simulink model "ekffede"  (Simulink 7.7)
settings: Solver=ode3  StartTime=0.0  StopTime=200  FixedStep=0.01  RelTol=1e-3
undefined symbols (not defined in the file): aerosimlib, Earth, WGS, WMM
libraries: simulink x15, aerolibconvert2 x4, aerolibtransform2 x2, aerolibgravity2 x2, aerolib6dof2 x1
settings Model: Creator="Fabrizio  Giulietti"  LastModifiedBy=Fede
settings OptimizationCC: InitFltsAndDblsToZero=on  OptimizeModelRefInitCode=on  LifeSpan=1
settings DebuggingCC: StrictBusMsg=Warning
settings HardwareCC: ProdLargestAtomicInteger=Long  ProdLargestAtomicFloat=Float  ProdEndianess=LittleEndian  ProdHWDeviceType=ARM Compatible->ARM 9
settings SFSimCC: SimParseCustomCode=off
settings RTWCC: SystemTargetFile=ert.tlc  TemplateMakefile=ert_default_tmf  Description=Embedded Coder  ProcessScript=ert_make_rtw_hook  RTWCompilerOptimization=On
settings CodeAppCC: IgnoreCustomStorageClasses=off
settings ERTTargetCC: FunctionExecutionProfile=off  MultiwordLength=2048  GenerateSampleERTMain=on  ERTCustomFileTemplate=example_file_process.tlc  ConvertIfToSwitch=off

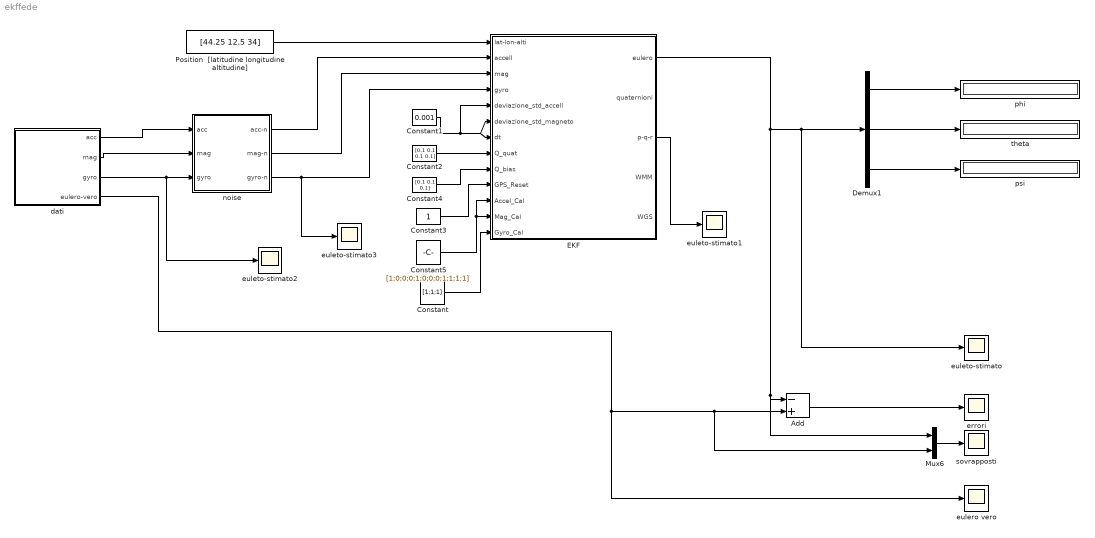
== system ekffede ==
  Add : Sum  Inputs=-+
  Constant : Constant  Value=[1;1;1]
  Constant1 : Constant  Value=0.001
  Constant2 : Constant  Value=[0.1 0.1 0.1 0.1]
  Constant3 : Constant
  Constant4 : Constant  Value=[0.1 0.1 0.1]
  Constant5 : Constant  Value=[1;0;0;0;1;0;0;0;1;1;1;1]
  Demux1 : Demux  Outputs=3
  EKF : Subsystem
  Mux6 : Mux  Inputs=2
  Position  [latitudine longitudine altitudine] : Constant  Value=[44.25 12.5 34]
  dati : Subsystem
  errori : Scope
      settings: YMin=-1.25  YMax=1.25
  eulero vero : Scope
      settings: SaveName=ScopeData15
  euleto-stimato{,1..3} (4 alike) : Scope
      euleto-stimato settings: YMin=-200  YMax=200  SaveName=ScopeData7
      euleto-stimato1 settings: YMin=-0.65  YMax=0.05  SaveName=ScopeData19
      euleto-stimato2 settings: SaveName=ScopeData20
      euleto-stimato3 settings: SaveName=ScopeData21
  noise : Subsystem  mask{bias_acc=|, bias_gyro=|, bias_mag=|, accel_noise_power=[0.0000, 0.0000, 0.0000], gyro_noise_power=[0.0000, 0.0000, 0.0000], mag_noise_power=[0.00000, 0.00000, 0.00000], acc_noise_freq=0.01, gyro_noise_freq=0.01, mag_noise_freq=0.01}
      mask bias_acc=|
      | [0  ;   0
      |  ;    0]
      mask bias_gyro=|
      | [0 ;   0
      |  ;    0]
      mask bias_mag=|
      | [0  ;   0
      |  ;    0]
      mask prompts: bias_acc "bias-acc"; bias_gyro "bias-gyro"; bias_mag "bias-mag"; accel_noise_power "accel-noise-power"; gyro_noise_power "gyro-noise-power"; mag_noise_power "mag-noise-power"; acc_noise_freq "acc-noise-freq"; gyro_noise_freq "gyro-noise-freq"; mag_noise_freq "mag-noise-freq"
  phi : Display
  psi : Display
  sovrapposti : Scope
      settings: TimeRange=200  YMin=-85  SaveName=ScopeData9
  theta : Display
  wires:
  Demux1/1 -> phi/1
  Demux1/2 -> theta/1
  Demux1/3 -> psi/1
  EKF/1(eulero) -> Demux1/1, euleto-stimato/1, Add/1, Mux6/1
  dati/4(eulero-vero) -> Add/2, Mux6/2, eulero vero/1
  Add/1 -> errori/1
  dati/2(mag) -> noise/2(mag)
  dati/3(gyro) -> noise/3(gyro), euleto-stimato2/1
  noise/2(mag-n) -> EKF/3(mag)
  Position  [latitudine longitudine altitudine]/1 -> EKF/1(lat-lon-alti)
  noise/3(gyro-n) -> EKF/4(gyro), euleto-stimato3/1
  noise/1(acc-n) -> EKF/2(accell)
  dati/1(acc) -> noise/1(acc)
  EKF/3(p-q-r) -> euleto-stimato1/1
  Constant1/1 -> EKF/5(deviazione_std_accell), EKF/6(deviazione_std_magneto), EKF/7(dt)
  Constant2/1 -> EKF/8(Q_quat)
  Constant4/1 -> EKF/9(Q_bias)
  Constant3/1 -> EKF/10(GPS_Reset)
  Mux6/1 -> sovrapposti/1
  Constant/1 -> EKF/13(Gyro_Cal)
  Constant5/1 -> EKF/11(Accel_Cal), EKF/12(Mag_Cal)

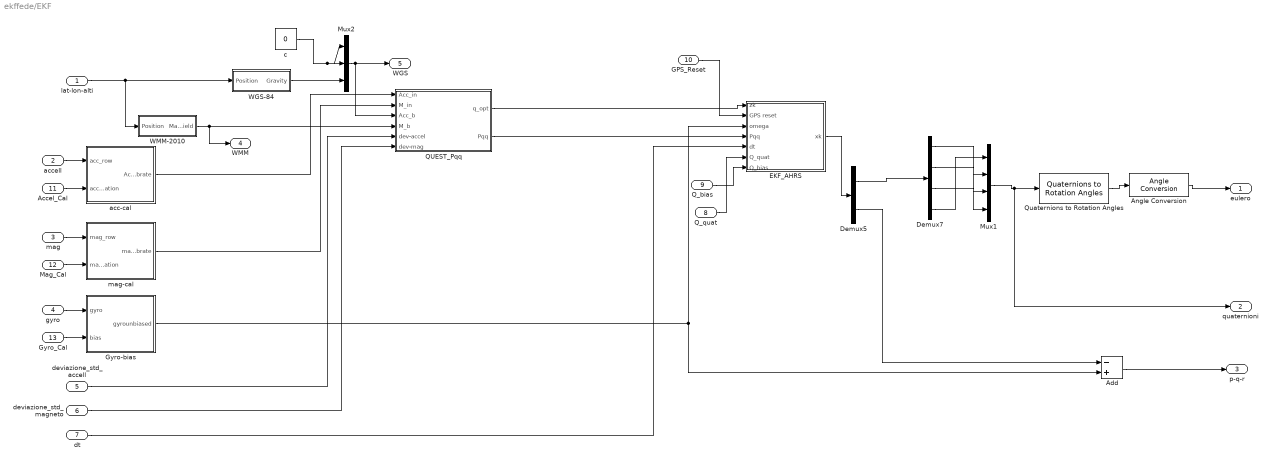
== system ekffede/EKF ==
  lat-lon-alti : Inport
  accell : Inport  Port=2  OutDataTypeStr=double
  mag : Inport  Port=3  OutDataTypeStr=double
  gyro : Inport  Port=4  OutDataTypeStr=double
  deviazione_std_accell : Inport  Port=5
  deviazione_std_magneto : Inport  Port=6
  dt : Inport  Port=7
  Q_quat : Inport  Port=8
  Q_bias : Inport  Port=9
  GPS_Reset : Inport  Port=10
  Accel_Cal : Inport  Port=11  OutDataTypeStr=double
  Mag_Cal : Inport  Port=12  OutDataTypeStr=double
  Gyro_Cal : Inport  Port=13  OutDataTypeStr=double
  Add : Sum  Inputs=-+
  Angle Conversion : aerolibconvert2/Angle Conversion  SystemSampleTime=-1  IU=rad  OU=deg
  Demux5 : Demux  Outputs=[4 3]
  Demux7 : Demux
  EKF_AHRS : Subsystem  mask{x0=[0 0 0 0 0 0 0]'}
      mask prompts: x0 "Initial condition vector"
  Gyro-bias : Stateflow chart  TreatAsAtomicUnit=on
  Mux1 : Mux
  Mux2 : Mux  Inputs=3
  QUEST_Pqq : Subsystem
  Quaternions to Rotation Angles : aerolibtransform2/Quaternions to Rotation Angles  SystemSampleTime=-1  rotationOrder=XYZ
  WGS-84 : Subsystem  AncestorBlock=aerosimlib/Earth/WGS-84
      mask Type: WGS-84 Earth model
      mask Description: The WGS-84 Earth model provides local Earth radii and gravity as a function of position.
      mask Help:
      | The block provides a WGS-84 geoid model of the Earth.
      | <P><B>Inputs:</B>
      | <LI>Position = current aircraft location [Latitude Longitude Altitude], in [rad rad m]</LI>
      | </P>
      | <P><B>Output:</B>
      | <LI>Rmeridian = the Earth meridian radius, in m</LI>
      | <LI>Rnormal = the Earth normal radius, in m</LI>
      | <LI>Re = the Earth equivalent radius, in m</LI>
      | <LI>Gravity = the normal gravity, in m/s^2</LI>
      | </P>
  WMM-2010 : Subsystem  AncestorBlock=aerosimlib/Earth/WMM-2000  mask(WMM-2000){wmmfile='C:\\Programmmi\\AeroSim\\wmm.cof', simdate=[26 05 2011]}
      mask prompts: wmmfile "WMM coefficient file:"; simdate "Simulation date [Day Month Year]:"
      mask help: The World Magnetic Model returns the Earth magnetic field components in body axes at current aircraft location.
      mask Help:
      | The block provides the magnetic field components at current aircraft location.
      | <P><B>Inputs:</B>
      | <LI>Position = the 3x1 vector of aircraft location [Latitude Longitude Altitude] in [rad rad m]</LI>
      | <LI>DCM = the frame transformation matrix from navigation to body frame</LI>
      | </P>
      | <P><B>Output:</B>
      | <LI>MagField = the 3x1 vector of magnetic field components in body axes</LI>
      | </P>
      | <P><B>Parameters:</B>
      | <LI>WMM coefficient file = the path to the WMM coefficient file, as a 'string'</LI>
      | <LI>Simulation date = the 1x3 vector of current date [Day Month Year]</LI>
      | </P>
  acc-cal : Stateflow chart  TreatAsAtomicUnit=on
  c : Constant  Value=0
  mag-cal : Stateflow chart  TreatAsAtomicUnit=on
  eulero : Outport
  quaternioni : Outport  Port=2
  p-q-r : Outport  Port=3
  WMM : Outport  Port=4
  WGS : Outport  Port=5
  wires:
  c/1 -> Mux2/1, Mux2/2
  Mux2/1 -> QUEST_Pqq/3(Acc_b), WGS/1
  lat-lon-alti/1 -> WMM-2010/1(Position), WGS-84/1(Position)
  GPS_Reset/1 -> EKF_AHRS/2(GPS reset)
  QUEST_Pqq/2(Pqq) -> EKF_AHRS/4(Pqq)
  Demux5/2 -> Add/1
  Quaternions to Rotation Angles/1 -> Angle Conversion/1
  WMM-2010/1(MagField) -> QUEST_Pqq/4(M_b), WMM/1
  WGS-84/1(Gravity) -> Mux2/3
  Angle Conversion/1 -> eulero/1
  Add/1 -> p-q-r/1
  deviazione_std_accell/1 -> QUEST_Pqq/5(dev-accel)
  deviazione_std_magneto/1 -> QUEST_Pqq/6(dev-mag)
  dt/1 -> EKF_AHRS/5(dt)
  EKF_AHRS/1(xk) -> Demux5/1
  Q_quat/1 -> EKF_AHRS/6(Q_quat)
  Q_bias/1 -> EKF_AHRS/7(Q_bias)
  Demux5/1 -> Demux7/1
  Mux1/1 -> Quaternions to Rotation Angles/1, quaternioni/1
  Demux7/4 -> Mux1/1
  Demux7/1 -> Mux1/2
  Demux7/2 -> Mux1/3
  Demux7/3 -> Mux1/4
  QUEST_Pqq/1(q_opt) -> EKF_AHRS/1(zk)
  Gyro-bias/1(gyrounbiased) -> EKF_AHRS/3(omega), Add/2
  Gyro_Cal/1 -> Gyro-bias/2(bias)
  gyro/1 -> Gyro-bias/1(gyro)
  accell/1 -> acc-cal/1(acc_row)
  acc-cal/1(Acc_calibrate) -> QUEST_Pqq/1(Acc_in)
  Accel_Cal/1 -> acc-cal/2(acc_calibration)
  Mag_Cal/1 -> mag-cal/2(mag_calibration)
  mag/1 -> mag-cal/1(mag_row)
  mag-cal/1(mag_calibrate) -> QUEST_Pqq/2(M_in)

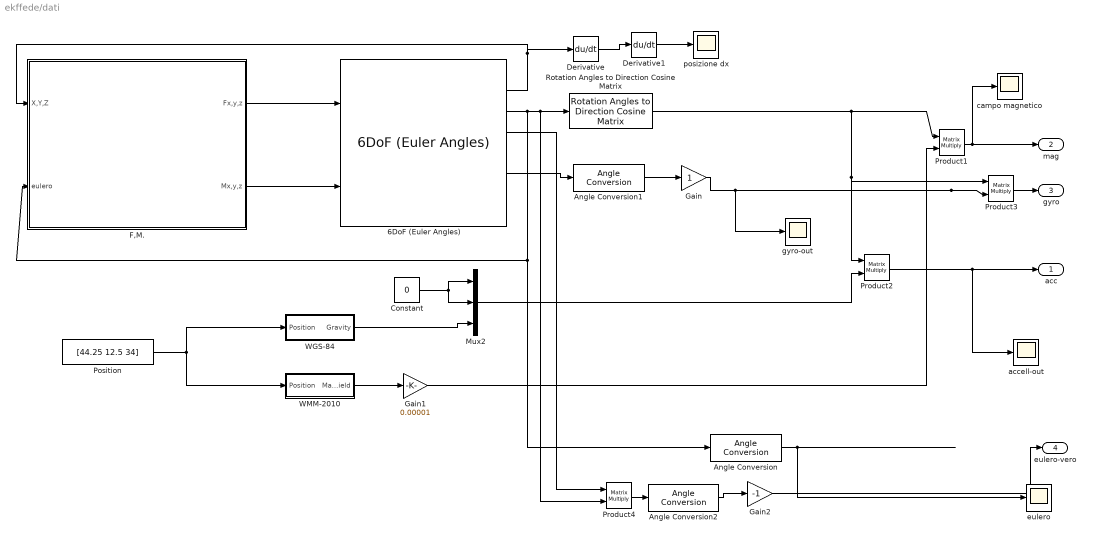
== system ekffede/dati ==
  6DoF (Euler Angles) : aerolib6dof2/6DoF (Euler Angles)  SystemSampleTime=-1  units=Metric (MKS)  mtype=Fixed  rep=Euler Angles  xme_0=[0 0 0]  Vm_0=[0 0 0]  eul_0=[0 0 0]  pm_0=[0 0 0]  mass_0=1000  mass_e=0.5  mass_f=2.0  inertia=eye(3)  inertia_e=eye(3)  inertia_f=2*eye(3)  k_quat=1.0
  Angle Conversion : aerolibconvert2/Angle Conversion  SystemSampleTime=-1  IU=rad  OU=deg
  Angle Conversion1 : aerolibconvert2/Angle Conversion  SystemSampleTime=-1  IU=rad  OU=rad
  Angle Conversion2 : aerolibconvert2/Angle Conversion  SystemSampleTime=-1  IU=rad  OU=deg
  Constant : Constant  Value=0
  Derivative : Derivative
  Derivative1 : Derivative
  F,M. : Subsystem  mask{rate_limiter_sfasamento=0.2, Fx=0, Fy=0, ampiezza_Fz=0.01, ampiezza_Fy=0, ampiezza_Fx=0, ampiezza_Mx=0.05, ampiezza_My=0.09, ampiezza_Mz=3.5, frequenza_Fz=0.01, frequenza_Fy=0.01, frequenza_Fx=0.01, frequenza_Mx=0.01, frequenza_My=0.01, frequenza_Mz=0.01, noise_power_sfasamento_m=0, sample_time_sfasamento_m=20, noise_power_m=0, noise_time_m=100, noise_power_F=0, noise_time_F=200, noise_power_sfasamento_F=0, sample_time_sfasamento_F=200}
      mask prompts: noise_power_sfasamento_F "sample_power_sfasamento_F"
  Gain : Gain
  Gain1 : Gain  Gain=0.00001
  Gain2 : Gain  Gain=-1
  Mux2 : Mux  Inputs=3
  Position : Constant  Value=[44.25 12.5 34]
  Product{1..4} (4 alike) : Product  Multiplication=Matrix(*)  RndMeth=Zero
  Rotation Angles to Direction Cosine Matrix : aerolibtransform2/Rotation Angles to Direction Cosine Matrix  SystemSampleTime=-1  rotationOrder=XYZ
  WGS-84 : Subsystem  AncestorBlock=aerosimlib/Earth/WGS-84
      mask Type: WGS-84 Earth model
      mask Description: The WGS-84 Earth model provides local Earth radii and gravity as a function of position.
      mask Help:
      | The block provides a WGS-84 geoid model of the Earth.
      | <P><B>Inputs:</B>
      | <LI>Position = current aircraft location [Latitude Longitude Altitude], in [rad rad m]</LI>
      | </P>
      | <P><B>Output:</B>
      | <LI>Rmeridian = the Earth meridian radius, in m</LI>
      | <LI>Rnormal = the Earth normal radius, in m</LI>
      | <LI>Re = the Earth equivalent radius, in m</LI>
      | <LI>Gravity = the normal gravity, in m/s^2</LI>
      | </P>
  WMM-2010 : Subsystem  AncestorBlock=aerosimlib/Earth/WMM-2000  mask(WMM-2000){wmmfile='C:\\Programmmi\\AeroSim\\wmm.cof', simdate=[26 05 2011]}
      mask prompts: wmmfile "WMM coefficient file:"; simdate "Simulation date [Day Month Year]:"
      mask help: The World Magnetic Model returns the Earth magnetic field components in body axes at current aircraft location.
      mask Help:
      | The block provides the magnetic field components at current aircraft location.
      | <P><B>Inputs:</B>
      | <LI>Position = the 3x1 vector of aircraft location [Latitude Longitude Altitude] in [rad rad m]</LI>
      | <LI>DCM = the frame transformation matrix from navigation to body frame</LI>
      | </P>
      | <P><B>Output:</B>
      | <LI>MagField = the 3x1 vector of magnetic field components in body axes</LI>
      | </P>
      | <P><B>Parameters:</B>
      | <LI>WMM coefficient file = the path to the WMM coefficient file, as a 'string'</LI>
      | <LI>Simulation date = the 1x3 vector of current date [Day Month Year]</LI>
      | </P>
  accell-out : Scope
      settings: SaveName=ScopeData24
  campo magnetico : Scope
      settings: SaveName=ScopeData6
  eulero : Scope
      settings: SaveName=ScopeData8
  gyro-out : Scope
      settings: SaveName=ScopeData3
  posizione dx : Scope
      settings: SaveName=ScopeData2
  acc : Outport
  mag : Outport  Port=2
  gyro : Outport  Port=3
  eulero-vero : Outport  Port=4
  wires:
  F,M./2(Mx,y,z) -> 6DoF (Euler Angles)/2
  6DoF (Euler Angles)/2 -> Derivative/1, F,M./1(X,Y,Z)
  F,M./1(Fx,y,z) -> 6DoF (Euler Angles)/1
  6DoF (Euler Angles)/3 -> F,M./2(eulero), Angle Conversion/1, Rotation Angles to Direction Cosine Matrix/1, Product4/2
  6DoF (Euler Angles)/6 -> Angle Conversion1/1
  Product1/1 -> campo magnetico/1, mag/1
  Mux2/1 -> Product2/2
  Angle Conversion/1 -> eulero/1
  Position/1 -> WMM-2010/1(Position), WGS-84/1(Position)
  WGS-84/1(Gravity) -> Mux2/3
  Constant/1 -> Mux2/1, Mux2/2
  Angle Conversion1/1 -> Gain/1
  WMM-2010/1(MagField) -> Gain1/1
  Gain1/1 -> Product1/2
  Derivative/1 -> Derivative1/1
  Derivative1/1 -> posizione dx/1
  Gain/1 -> gyro-out/1, Product3/2
  Product2/1 -> acc/1, accell-out/1
  Rotation Angles to Direction Cosine Matrix/1 -> Product1/1, Product2/1, Product3/1
  Product3/1 -> gyro/1
  Product4/1 -> Angle Conversion2/1
  Angle Conversion2/1 -> Gain2/1
  6DoF (Euler Angles)/4 -> Product4/1
  Gain2/1 -> eulero-vero/1

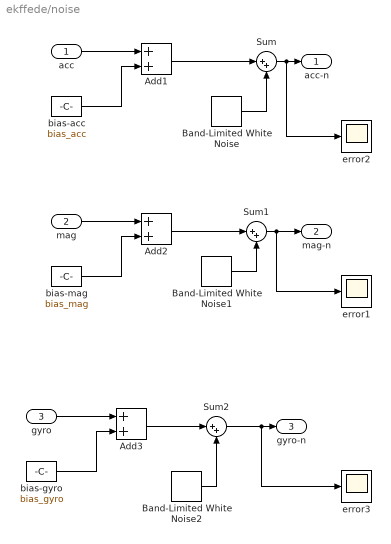
== system ekffede/noise ==
  acc : Inport
  mag : Inport  Port=2
  gyro : Inport  Port=3
  Add1 : Sum
  Add2 : Sum
  Add3 : Sum
  Band-Limited White Noise : simulink/Sources/Band-Limited White Noise  SystemSampleTime=-1  Cov=accel_noise_power  Ts=acc_noise_freq  seed=[23341]
  Band-Limited White Noise1 : simulink/Sources/Band-Limited White Noise  SystemSampleTime=-1  Cov=mag_noise_power  Ts=mag_noise_freq  seed=[23341]
  Band-Limited White Noise2 : simulink/Sources/Band-Limited White Noise  SystemSampleTime=-1  Cov=gyro_noise_power  Ts=gyro_noise_freq  seed=[23341]
  Sum : Sum  Inputs=|++
  Sum1 : Sum  Inputs=|++
  Sum2 : Sum  Inputs=|++
  bias-acc : Constant  Value=bias_acc
  bias-gyro : Constant  Value=bias_gyro
  bias-mag : Constant  Value=bias_mag
  error1 : Scope
      settings: YMin=-0.025  YMax=0.475  SaveName=ScopeData13
  error2 : Scope
      settings: SaveName=ScopeData12
  error3 : Scope
      settings: SaveName=ScopeData14
  acc-n : Outport
  mag-n : Outport  Port=2
  gyro-n : Outport  Port=3
  wires:
  gyro/1 -> Add3/1
  Sum2/1 -> error3/1, gyro-n/1
  Add3/1 -> Sum2/1
  bias-gyro/1 -> Add3/2
  mag/1 -> Add2/1
  bias-mag/1 -> Add2/2
  acc/1 -> Add1/1
  Sum/1 -> error2/1, acc-n/1
  Add1/1 -> Sum/1
  bias-acc/1 -> Add1/2
  Band-Limited White Noise/1 -> Sum/2
  Band-Limited White Noise2/1 -> Sum2/2
  Add2/1 -> Sum1/1
  Band-Limited White Noise1/1 -> Sum1/2
  Sum1/1 -> mag-n/1, error1/1

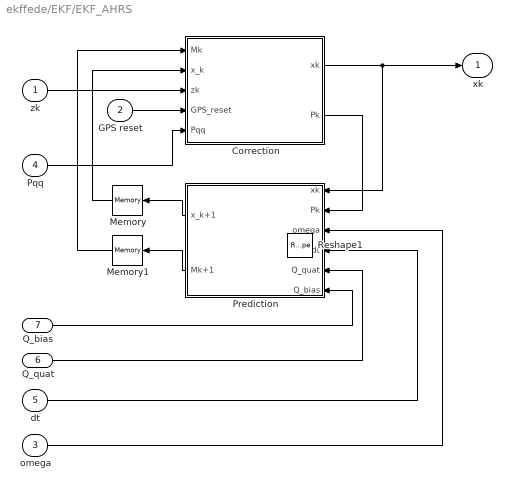
== system ekffede/EKF/EKF_AHRS ==
  zk : Inport
  GPS reset : Inport  Port=2
  omega : Inport  Port=3
  Pqq : Inport  Port=4
  dt : Inport  Port=5
  Q_quat : Inport  Port=6
  Q_bias : Inport  Port=7
  Correction : Subsystem  TreatAsAtomicUnit=on
  Memory : Memory  X0=x0
  Memory1 : Memory  X0=diag([ones(4,1)*0.003;zeros(3,1)])
  Prediction : Subsystem  TreatAsAtomicUnit=on
  Reshape1 : Reshape
  xk : Outport
  wires:
  GPS reset/1 -> Correction/4(GPS_reset)
  Memory1/1 -> Correction/1(Mk)
  Prediction/2(Mk+1) -> Memory1/1
  Memory/1 -> Correction/2(x_k)
  Prediction/1(x_k+1) -> Memory/1
  zk/1 -> Correction/3(zk)
  Correction/2(Pk) -> Prediction/2(Pk)
  Correction/1(xk) -> Prediction/1(xk), xk/1
  omega/1 -> Prediction/3(omega)
  Pqq/1 -> Correction/5(Pqq)
  dt/1 -> Prediction/4(dt)
  Q_bias/1 -> Prediction/6(Q_bias)
  Q_quat/1 -> Prediction/5(Q_quat)

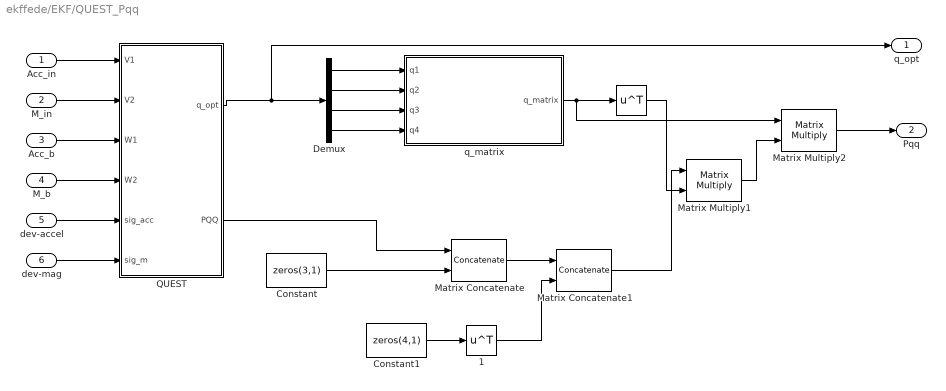
== system ekffede/EKF/QUEST_Pqq ==
  Acc_in : Inport
  M_in : Inport  Port=2
  Acc_b : Inport  Port=3
  M_b : Inport  Port=4
  dev-accel : Inport  Port=5
  dev-mag : Inport  Port=6
  " " : Math  Operator=transpose  SaturateOnIntegerOverflow=on
  " 1" : Math  Operator=transpose  SaturateOnIntegerOverflow=on
  Constant : Constant  Value=zeros(3,1)
  Constant1 : Constant  Value=zeros(4,1)
  Demux : Demux
  Matrix Concatenate : Concatenate  Mode=Multidimensional array  ConcatenateDimension=2
  Matrix Concatenate1 : Concatenate  Mode=Multidimensional array
  Matrix Multiply1 : Product  Multiplication=Matrix(*)
  Matrix Multiply2 : Product  Multiplication=Matrix(*)
  QUEST : Stateflow chart  TreatAsAtomicUnit=on
  q_matrix : Stateflow chart  TreatAsAtomicUnit=on
  q_opt : Outport
  Pqq : Outport  Port=2
  wires:
  QUEST/1(q_opt) -> Demux/1, q_opt/1
  QUEST/2(PQQ) -> Matrix Concatenate/1
  Constant/1 -> Matrix Concatenate/2
  Matrix Concatenate/1 -> Matrix Concatenate1/1
  Constant1/1 -> " 1"/1
  Demux/1 -> q_matrix/1(q1)
  Demux/2 -> q_matrix/2(q2)
  Demux/3 -> q_matrix/3(q3)
  Demux/4 -> q_matrix/4(q4)
  M_in/1 -> QUEST/2(V2)
  q_matrix/1(q_matrix) -> " "/1, Matrix Multiply2/1
  Acc_b/1 -> QUEST/3(W1)
  M_b/1 -> QUEST/4(W2)
  Matrix Concatenate1/1 -> Matrix Multiply1/1
  " "/1 -> Matrix Multiply1/2
  Matrix Multiply1/1 -> Matrix Multiply2/2
  Matrix Multiply2/1 -> Pqq/1
  dev-accel/1 -> QUEST/5(sig_acc)
  " 1"/1 -> Matrix Concatenate1/2
  Acc_in/1 -> QUEST/1(V1)
  dev-mag/1 -> QUEST/6(sig_m)

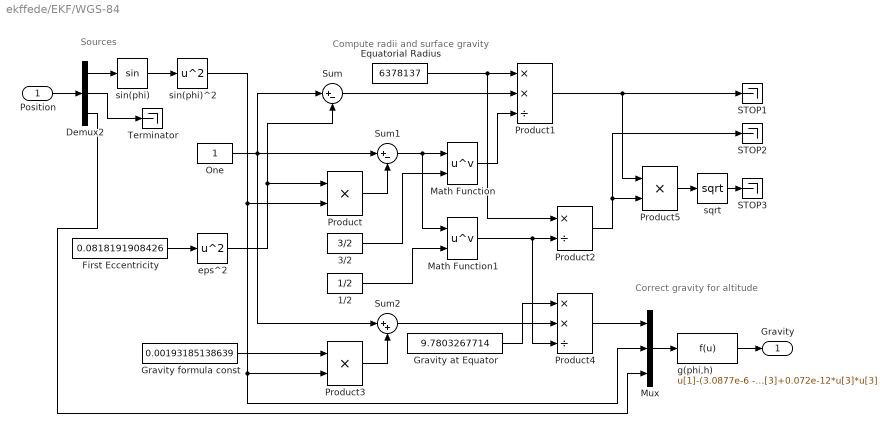
== system ekffede/EKF/WGS-84 ==
  note: Correct gravity for altitude
  note: Compute radii and surface gravity
  note: Sources
  Position : Inport
  1/2 : Constant  Value=1/2
  3/2 : Constant  Value=3/2
  Demux2 : Demux  Outputs=3
  Equatorial Radius : Constant  Value=6378137
  First Eccentricity : Constant  Value=0.0818191908426
  Gravity at Equator : Constant  Value=9.7803267714
  Gravity formula const : Constant  Value=0.00193185138639
  Math Function : Math  Operator=pow  SaturateOnIntegerOverflow=on
  Math Function1 : Math  Operator=pow  SaturateOnIntegerOverflow=on
  Mux : Mux  Inputs=3
  One : Constant
  Product : Product  SaturateOnIntegerOverflow=on  InputSameDT=on  OutDataTypeStr=Inherit: Same as first input
  Product1 : Product  Inputs=**/  SaturateOnIntegerOverflow=on  InputSameDT=on  OutDataTypeStr=Inherit: Same as first input
  Product2 : Product  Inputs=*/  SaturateOnIntegerOverflow=on  InputSameDT=on  OutDataTypeStr=Inherit: Same as first input
  Product3 : Product  SaturateOnIntegerOverflow=on  InputSameDT=on  OutDataTypeStr=Inherit: Same as first input
  Product4 : Product  Inputs=**/  SaturateOnIntegerOverflow=on  InputSameDT=on  OutDataTypeStr=Inherit: Same as first input
  Product5 : Product  SaturateOnIntegerOverflow=on  InputSameDT=on  OutDataTypeStr=Inherit: Same as first input
  STOP1 : Terminator
  STOP2 : Terminator
  STOP3 : Terminator
  Sum : Sum  Inputs=|+-  SaturateOnIntegerOverflow=on  InputSameDT=on  OutDataTypeStr=Inherit: Same as first input
  Sum1 : Sum  Inputs=|+-  SaturateOnIntegerOverflow=on  InputSameDT=on  OutDataTypeStr=Inherit: Same as first input
  Sum2 : Sum  Inputs=|++  SaturateOnIntegerOverflow=on  InputSameDT=on  OutDataTypeStr=Inherit: Same as first input
  Terminator : Terminator
  eps^2 : Math  Operator=square  SaturateOnIntegerOverflow=on
  g(phi,h) : Fcn  Expr=u[1]-(3.0877e-6 - 0.0044e-6*u[2])*u[3]+0.072e-12*u[3]*u[3]
  sin(phi) : Trigonometry
  sin(phi)^2 : Math  Operator=square  SaturateOnIntegerOverflow=on
  sqrt : Math  Operator=sqrt  SaturateOnIntegerOverflow=on
  Gravity : Outport
  wires:
  Demux2/3 -> Mux/3
  g(phi,h)/1 -> Gravity/1
  Mux/1 -> g(phi,h)/1
  Demux2/2 -> Terminator/1
  Demux2/1 -> sin(phi)/1
  Position/1 -> Demux2/1
  Product4/1 -> Mux/1
  Sum2/1 -> Product4/2
  Gravity at Equator/1 -> Product4/1
  Product3/1 -> Sum2/2
  Gravity formula const/1 -> Product3/1
  Product2/1 -> Product5/2, STOP2/1
  Product1/1 -> Product5/1, STOP1/1
  Math Function1/1 -> Product4/3, Product2/2
  Math Function/1 -> Product1/3
  Sum/1 -> Product1/2
  Equatorial Radius/1 -> Product2/1, Product1/1
  1/2/1 -> Math Function1/2
  3/2/1 -> Math Function/2
  Sum1/1 -> Math Function1/1, Math Function/1
  Product/1 -> Sum1/2
  One/1 -> Sum/1, Sum2/1, Sum1/1
  sin(phi)^2/1 -> Mux/2, Product3/2, Product/2
  sin(phi)/1 -> sin(phi)^2/1
  eps^2/1 -> Product/1, Sum/2
  First Eccentricity/1 -> eps^2/1
  Product5/1 -> sqrt/1
  sqrt/1 -> STOP3/1

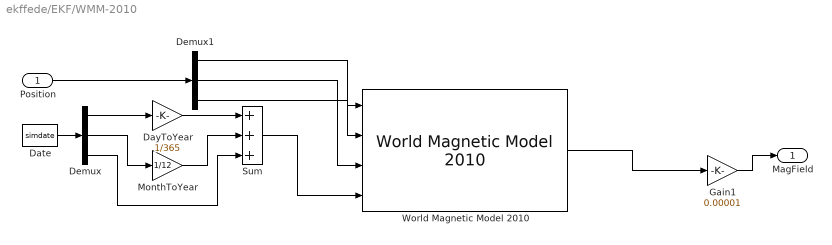
== system ekffede/EKF/WMM-2010 ==
  Position : Inport  OutDataTypeStr=double  PortDimensions=[3 1]
  Date : Constant  Value=simdate
  DayToYear : Gain  Gain=1/365  SaturateOnIntegerOverflow=on  OutDataTypeStr=Inherit: Same as input  ParamDataTypeStr=Inherit: Same as input
  Demux : Demux  Outputs=3
  Demux1 : Demux  Outputs=3
  Gain1 : Gain  Gain=0.00001
  MonthToYear : Gain  Gain=1/12  SaturateOnIntegerOverflow=on  OutDataTypeStr=Inherit: Same as input  ParamDataTypeStr=Inherit: Same as input
  Sum : Sum  Inputs=+++  SaturateOnIntegerOverflow=on  InputSameDT=on  OutDataTypeStr=Inherit: Same as first input
  World Magnetic Model 2010 : aerolibgravity2/World Magnetic Model 2010  SystemSampleTime=-1  units=Metric (MKS)  time_in=on  month=January  day=1  year=2010  action=Error  h_out=off  dec_out=off  inc_out=off  ti_out=off
  MagField : Outport
  wires:
  Sum/1 -> World Magnetic Model 2010/4
  MonthToYear/1 -> Sum/2
  Demux/3 -> Sum/3
  Demux/2 -> MonthToYear/1
  DayToYear/1 -> Sum/1
  Demux/1 -> DayToYear/1
  Date/1 -> Demux/1
  Position/1 -> Demux1/1
  Demux1/1 -> World Magnetic Model 2010/2
  Demux1/2 -> World Magnetic Model 2010/3
  Demux1/3 -> World Magnetic Model 2010/1
  Gain1/1 -> MagField/1
  World Magnetic Model 2010/1 -> Gain1/1

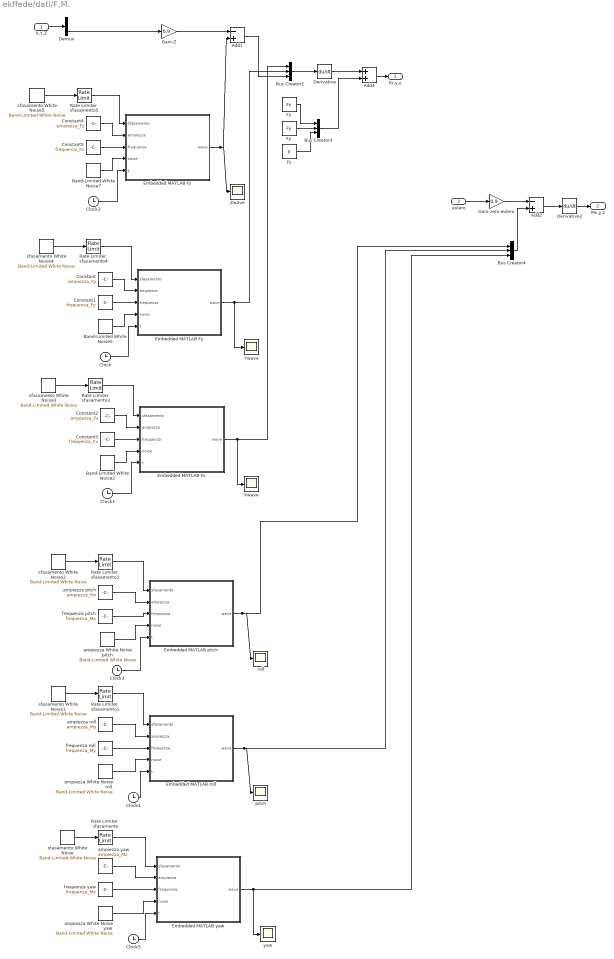
== system ekffede/dati/F,M. ==
  X,Y,Z : Inport
  eulero : Inport  Port=2
  Add1 : Sum  Inputs=-+
  Add2 : Sum  Inputs=-+
  Add4 : Sum
  Band-Limited White Noise2 : simulink/Sources/Band-Limited White Noise  SystemSampleTime=-1  Cov=noise_power_F  Ts=0.01  seed=[23341]
  Band-Limited White Noise5 : simulink/Sources/Band-Limited White Noise  SystemSampleTime=-1  Cov=noise_power_F  Ts=0.01  seed=[23341]
  Band-Limited White Noise7 : simulink/Sources/Band-Limited White Noise  SystemSampleTime=-1  Cov=noise_power_F  Ts=0.01  seed=[23341]
  Bus Creator2 : BusCreator  Inputs=3
  Bus Creator3 : BusCreator  Inputs=3
  Bus Creator4 : BusCreator  Inputs=3
  Clock{,1..5} (6 alike) : Clock
      settings: Decimation=10
  Constant : Constant  Value=ampiezza_Fy
  Constant1 : Constant  Value=frequenza_Fy
  Constant2 : Constant  Value=ampiezza_Fx
  Constant3 : Constant  Value=frequenza_Fx
  Constant4 : Constant  Value=ampiezza_Fz
  Constant5 : Constant  Value=frequenza_Fz
  Demux : Demux  Outputs=3
  Derivative : Derivative
  Derivative2 : Derivative
  Embedded MATLAB Fx : Stateflow chart  TreatAsAtomicUnit=on
  Embedded MATLAB Fy : Stateflow chart  TreatAsAtomicUnit=on
  Embedded MATLAB Fz : Stateflow chart  TreatAsAtomicUnit=on
  Embedded MATLAB pitch : Stateflow chart  TreatAsAtomicUnit=on
  Embedded MATLAB roll : Stateflow chart  TreatAsAtomicUnit=on
  Embedded MATLAB yaw : Stateflow chart  TreatAsAtomicUnit=on
  Fx : Constant  Value=Fx
  Fy : Constant  Value=Fy
  Fz : Constant  Value=0
  Gain-Z : Gain  Gain=0.9
  Gain-zero eulero : Gain  Gain=0.9
  Rate Limiter  sfasamento{,1..5} (6 alike) : RateLimiter  RisingSlewLimit=rate_limiter_sfasamento  FallingSlewLimit=-rate_limiter_sfasamento  SampleTimeMode=inherited
  Xwave : Scope
      settings: YMin=0.00010125  YMax=0.00010425  SaveName=ScopeData3
  Ywave : Scope
      settings: YMin=9.525e-005  YMax=9.775e-005  SaveName=ScopeData11
  Zwave : Scope
      settings: YMin=8.775e-005  YMax=9.3e-005  SaveName=ScopeData4
  ampiezza White Noise pitch : simulink/Sources/Band-Limited White Noise  SystemSampleTime=-1  Cov=noise_power_m  Ts=0.01  seed=[23341]
  ampiezza White Noise roll : simulink/Sources/Band-Limited White Noise  SystemSampleTime=-1  Cov=noise_power_m  Ts=0.01  seed=[23341]
  ampiezza White Noise yaw : simulink/Sources/Band-Limited White Noise  SystemSampleTime=-1  Cov=noise_power_m  Ts=0.01  seed=[23341]
  ampiezza pitch : Constant  Value=ampiezza_Mx
  ampiezza roll : Constant  Value=ampiezza_My
  ampiezza yaw : Constant  Value=ampiezza_Mz
  frequenza pitch : Constant  Value=frequenza_Mx
  frequenza roll : Constant  Value=frequenza_My
  frequenza yaw : Constant  Value=frequenza_Mz
  pitch : Scope
      settings: YMin=0.06005  YMax=0.06095  SaveName=ScopeData10
  roll : Scope
      settings: YMin=0.0525  YMax=0.05675  SaveName=ScopeData5
  sfasamento White Noise : simulink/Sources/Band-Limited White Noise  SystemSampleTime=-1  Cov=noise_power_sfasamento_m  Ts=0.01  seed=[23341]
  sfasamento White Noise1 : simulink/Sources/Band-Limited White Noise  SystemSampleTime=-1  Cov=noise_power_sfasamento_m  Ts=0.01  seed=[23341]
  sfasamento White Noise2 : simulink/Sources/Band-Limited White Noise  SystemSampleTime=-1  Cov=noise_power_sfasamento_m  Ts=0.01  seed=[23341]
  sfasamento White Noise3 : simulink/Sources/Band-Limited White Noise  SystemSampleTime=-1  Cov=noise_power_sfasamento_F  Ts=0.01  seed=[23341]
  sfasamento White Noise4 : simulink/Sources/Band-Limited White Noise  SystemSampleTime=-1  Cov=noise_power_sfasamento_F  Ts=0.01  seed=[23341]
  sfasamento White Noise5 : simulink/Sources/Band-Limited White Noise  SystemSampleTime=-1  Cov=noise_power_sfasamento_F  Ts=0.01  seed=[23341]
  yaw : Scope
      settings: YMin=0.0626  YMax=0.0639  SaveName=ScopeData17
  Fx,y,z : Outport
  Mx,y,z : Outport  Port=2
  wires:
  Derivative/1 -> Add4/1
  Gain-Z/1 -> Add1/1
  Demux/3 -> Gain-Z/1
  Add1/1 -> Bus Creator2/3
  Bus Creator2/1 -> Derivative/1
  Constant1/1 -> Embedded MATLAB Fy/3(frequenza)
  Embedded MATLAB Fy/1(wave) -> Ywave/1, Bus Creator2/2
  Clock/1 -> Embedded MATLAB Fy/5(t)
  Band-Limited White Noise5/1 -> Embedded MATLAB Fy/4(noise)
  Constant3/1 -> Embedded MATLAB Fx/3(frequenza)
  Embedded MATLAB Fx/1(wave) -> Xwave/1, Bus Creator2/1
  Clock1/1 -> Embedded MATLAB Fx/5(t)
  Band-Limited White Noise2/1 -> Embedded MATLAB Fx/4(noise)
  Constant5/1 -> Embedded MATLAB Fz/3(frequenza)
  Embedded MATLAB Fz/1(wave) -> Zwave/1, Add1/2
  Clock2/1 -> Embedded MATLAB Fz/5(t)
  Band-Limited White Noise7/1 -> Embedded MATLAB Fz/4(noise)
  Fx/1 -> Bus Creator3/1
  Fy/1 -> Bus Creator3/2
  Fz/1 -> Bus Creator3/3
  Bus Creator3/1 -> Add4/2
  Embedded MATLAB pitch/1(wave) -> roll/1, Bus Creator4/1
  X,Y,Z/1 -> Demux/1
  Add4/1 -> Fx,y,z/1
  Constant4/1 -> Embedded MATLAB Fz/2(ampiezza)
  Constant/1 -> Embedded MATLAB Fy/2(ampiezza)
  Constant2/1 -> Embedded MATLAB Fx/2(ampiezza)
  frequenza roll/1 -> Embedded MATLAB roll/3(frequenza)
  ampiezza roll/1 -> Embedded MATLAB roll/2(ampiezza)
  Embedded MATLAB roll/1(wave) -> pitch/1, Bus Creator4/2
  ampiezza White Noise roll/1 -> Embedded MATLAB roll/4(noise)
  frequenza yaw/1 -> Embedded MATLAB yaw/3(frequenza)
  ampiezza yaw/1 -> Embedded MATLAB yaw/2(ampiezza)
  Embedded MATLAB yaw/1(wave) -> yaw/1, Bus Creator4/3
  ampiezza White Noise yaw/1 -> Embedded MATLAB yaw/4(noise)
  Gain-zero eulero/1 -> Add2/1
  eulero/1 -> Gain-zero eulero/1
  Bus Creator4/1 -> Add2/2
  Add2/1 -> Derivative2/1
  Derivative2/1 -> Mx,y,z/1
  sfasamento White Noise/1 -> Rate Limiter  sfasamento/1
  Rate Limiter  sfasamento/1 -> Embedded MATLAB yaw/1(sfasamento)
  sfasamento White Noise1/1 -> Rate Limiter  sfasamento1/1
  Rate Limiter  sfasamento1/1 -> Embedded MATLAB roll/1(sfasamento)
  frequenza pitch/1 -> Embedded MATLAB pitch/3(frequenza)
  ampiezza pitch/1 -> Embedded MATLAB pitch/2(ampiezza)
  Clock3/1 -> Embedded MATLAB pitch/5(t)
  ampiezza White Noise pitch/1 -> Embedded MATLAB pitch/4(noise)
  sfasamento White Noise2/1 -> Rate Limiter  sfasamento2/1
  Rate Limiter  sfasamento2/1 -> Embedded MATLAB pitch/1(sfasamento)
  sfasamento White Noise3/1 -> Rate Limiter  sfasamento3/1
  Rate Limiter  sfasamento3/1 -> Embedded MATLAB Fx/1(sfasamento)
  sfasamento White Noise4/1 -> Rate Limiter  sfasamento4/1
  Rate Limiter  sfasamento4/1 -> Embedded MATLAB Fy/1(sfasamento)
  sfasamento White Noise5/1 -> Rate Limiter  sfasamento5/1
  Rate Limiter  sfasamento5/1 -> Embedded MATLAB Fz/1(sfasamento)
  Clock5/1 -> Embedded MATLAB yaw/5(t)
  Clock4/1 -> Embedded MATLAB roll/5(t)

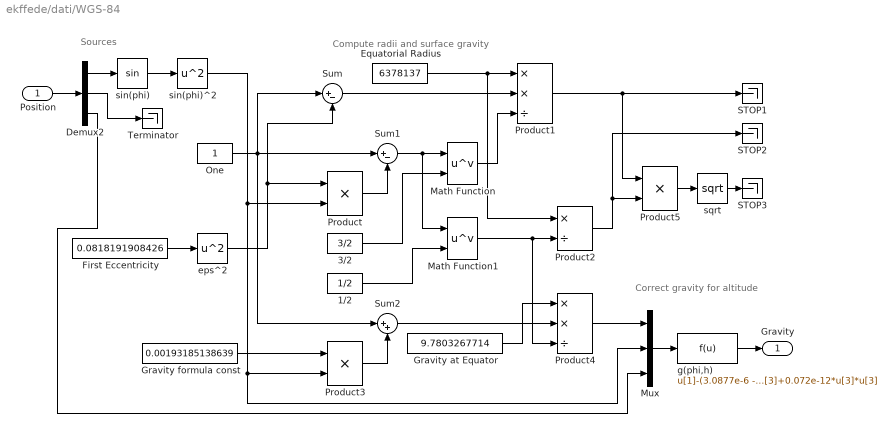
== system ekffede/dati/WGS-84 ==
  note: Correct gravity for altitude
  note: Compute radii and surface gravity
  note: Sources
  Position : Inport
  1/2 : Constant  Value=1/2
  3/2 : Constant  Value=3/2
  Demux2 : Demux  Outputs=3
  Equatorial Radius : Constant  Value=6378137
  First Eccentricity : Constant  Value=0.0818191908426
  Gravity at Equator : Constant  Value=9.7803267714
  Gravity formula const : Constant  Value=0.00193185138639
  Math Function : Math  Operator=pow  SaturateOnIntegerOverflow=on
  Math Function1 : Math  Operator=pow  SaturateOnIntegerOverflow=on
  Mux : Mux  Inputs=3
  One : Constant
  Product : Product  SaturateOnIntegerOverflow=on  InputSameDT=on  OutDataTypeStr=Inherit: Same as first input
  Product1 : Product  Inputs=**/  SaturateOnIntegerOverflow=on  InputSameDT=on  OutDataTypeStr=Inherit: Same as first input
  Product2 : Product  Inputs=*/  SaturateOnIntegerOverflow=on  InputSameDT=on  OutDataTypeStr=Inherit: Same as first input
  Product3 : Product  SaturateOnIntegerOverflow=on  InputSameDT=on  OutDataTypeStr=Inherit: Same as first input
  Product4 : Product  Inputs=**/  SaturateOnIntegerOverflow=on  InputSameDT=on  OutDataTypeStr=Inherit: Same as first input
  Product5 : Product  SaturateOnIntegerOverflow=on  InputSameDT=on  OutDataTypeStr=Inherit: Same as first input
  STOP1 : Terminator
  STOP2 : Terminator
  STOP3 : Terminator
  Sum : Sum  Inputs=|+-  SaturateOnIntegerOverflow=on  InputSameDT=on  OutDataTypeStr=Inherit: Same as first input
  Sum1 : Sum  Inputs=|+-  SaturateOnIntegerOverflow=on  InputSameDT=on  OutDataTypeStr=Inherit: Same as first input
  Sum2 : Sum  Inputs=|++  SaturateOnIntegerOverflow=on  InputSameDT=on  OutDataTypeStr=Inherit: Same as first input
  Terminator : Terminator
  eps^2 : Math  Operator=square  SaturateOnIntegerOverflow=on
  g(phi,h) : Fcn  Expr=u[1]-(3.0877e-6 - 0.0044e-6*u[2])*u[3]+0.072e-12*u[3]*u[3]
  sin(phi) : Trigonometry
  sin(phi)^2 : Math  Operator=square  SaturateOnIntegerOverflow=on
  sqrt : Math  Operator=sqrt  SaturateOnIntegerOverflow=on
  Gravity : Outport
  wires:
  Demux2/3 -> Mux/3
  g(phi,h)/1 -> Gravity/1
  Mux/1 -> g(phi,h)/1
  Demux2/2 -> Terminator/1
  Demux2/1 -> sin(phi)/1
  Position/1 -> Demux2/1
  Product4/1 -> Mux/1
  Sum2/1 -> Product4/2
  Gravity at Equator/1 -> Product4/1
  Product3/1 -> Sum2/2
  Gravity formula const/1 -> Product3/1
  Product2/1 -> Product5/2, STOP2/1
  Product1/1 -> Product5/1, STOP1/1
  Math Function1/1 -> Product4/3, Product2/2
  Math Function/1 -> Product1/3
  Sum/1 -> Product1/2
  Equatorial Radius/1 -> Product2/1, Product1/1
  1/2/1 -> Math Function1/2
  3/2/1 -> Math Function/2
  Sum1/1 -> Math Function1/1, Math Function/1
  Product/1 -> Sum1/2
  One/1 -> Sum/1, Sum2/1, Sum1/1
  sin(phi)^2/1 -> Mux/2, Product3/2, Product/2
  sin(phi)/1 -> sin(phi)^2/1
  eps^2/1 -> Product/1, Sum/2
  First Eccentricity/1 -> eps^2/1
  Product5/1 -> sqrt/1
  sqrt/1 -> STOP3/1

== system ekffede/dati/WMM-2010 ==
  Position : Inport  OutDataTypeStr=double  PortDimensions=[3 1]
  Date : Constant  Value=simdate
  DayToYear : Gain  Gain=1/365  SaturateOnIntegerOverflow=on  OutDataTypeStr=Inherit: Same as input  ParamDataTypeStr=Inherit: Same as input
  Demux : Demux  Outputs=3
  Demux1 : Demux  Outputs=3
  MonthToYear : Gain  Gain=1/12  SaturateOnIntegerOverflow=on  OutDataTypeStr=Inherit: Same as input  ParamDataTypeStr=Inherit: Same as input
  Sum : Sum  Inputs=+++  SaturateOnIntegerOverflow=on  InputSameDT=on  OutDataTypeStr=Inherit: Same as first input
  World Magnetic Model 2010 : aerolibgravity2/World Magnetic Model 2010  SystemSampleTime=-1  units=Metric (MKS)  time_in=on  month=January  day=1  year=2010  action=Error  h_out=off  dec_out=off  inc_out=off  ti_out=off
  MagField : Outport
  wires:
  Sum/1 -> World Magnetic Model 2010/4
  MonthToYear/1 -> Sum/2
  Demux/3 -> Sum/3
  Demux/2 -> MonthToYear/1
  DayToYear/1 -> Sum/1
  Demux/1 -> DayToYear/1
  Date/1 -> Demux/1
  World Magnetic Model 2010/1 -> MagField/1
  Position/1 -> Demux1/1
  Demux1/1 -> World Magnetic Model 2010/2
  Demux1/2 -> World Magnetic Model 2010/3
  Demux1/3 -> World Magnetic Model 2010/1

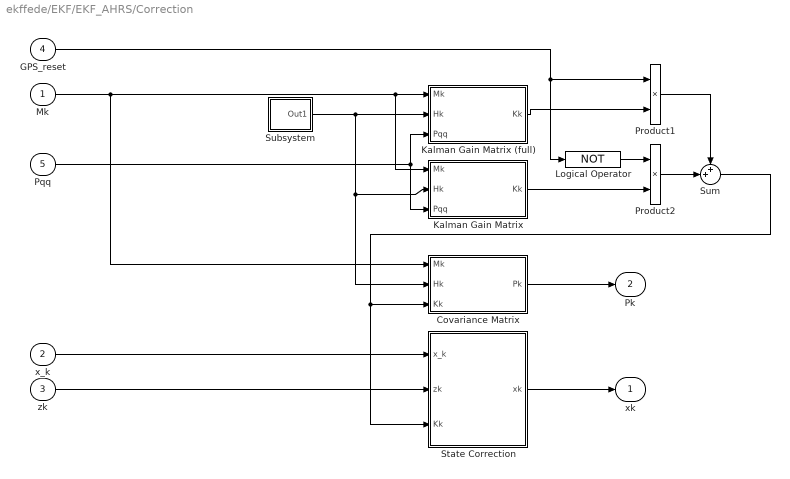
== system ekffede/EKF/EKF_AHRS/Correction ==
  Mk : Inport
  x_k : Inport  Port=2
  zk : Inport  Port=3
  GPS_reset : Inport  Port=4
  Pqq : Inport  Port=5
  Covariance Matrix : Subsystem
  Kalman Gain Matrix : Subsystem
  Kalman Gain Matrix (full) : Subsystem
  Logical Operator : Logic  Operator=NOT  AllPortsSameDT=off  OutDataTypeStr=boolean
  Product1 : Product  RndMeth=Zero
  Product2 : Product  RndMeth=Zero
  State Correction : Subsystem
  Subsystem : Subsystem
      mask Display: disp('h')
  Sum : Sum  Inputs=++|
  xk : Outport
  Pk : Outport  Port=2
  wires:
  Sum/1 -> State Correction/3(Kk), Covariance Matrix/3(Kk)
  Product1/1 -> Sum/1
  Product2/1 -> Sum/2
  Logical Operator/1 -> Product2/1
  Kalman Gain Matrix/1(Kk) -> Product2/2
  GPS_reset/1 -> Logical Operator/1, Product1/1
  Kalman Gain Matrix (full)/1(Kk) -> Product1/2
  Mk/1 -> Covariance Matrix/1(Mk), Kalman Gain Matrix (full)/1(Mk), Kalman Gain Matrix/1(Mk)
  x_k/1 -> State Correction/1(x_k)
  Subsystem/1(Out1) -> Covariance Matrix/2(Hk), Kalman Gain Matrix/2(Hk), Kalman Gain Matrix (full)/2(Hk)
  zk/1 -> State Correction/2(zk)
  Covariance Matrix/1(Pk) -> Pk/1
  State Correction/1(xk) -> xk/1
  Pqq/1 -> Kalman Gain Matrix (full)/3(Pqq), Kalman Gain Matrix/3(Pqq)

== system ekffede/EKF/EKF_AHRS/Prediction ==
  xk : Inport
  Pk : Inport  Port=2
  omega : Inport  Port=3
  dt : Inport  Port=4
  Q_quat : Inport  Port=5
  Q_bias : Inport  Port=6
  Prediction : Subsystem
  x_k+1 : Outport
  Mk+1 : Outport  Port=2
  wires:
  Prediction/2(Mk+1) -> Mk+1/1
  Prediction/1(x_k+1) -> x_k+1/1
  xk/1 -> Prediction/1(xk)
  Pk/1 -> Prediction/2(Pk)
  omega/1 -> Prediction/3(omega)
  dt/1 -> Prediction/4(dt)
  Q_quat/1 -> Prediction/5(Q_quat)
  Q_bias/1 -> Prediction/6(Q_bias)

== system ekffede/EKF/EKF_AHRS/Correction/Covariance Matrix ==
  Mk : Inport
  Hk : Inport  Port=2
  Kk : Inport  Port=3
  Constant : Constant  Value=eye(7)
  Product1 : Product  Multiplication=Matrix(*)  RndMeth=Zero
  Product3 : Product  Multiplication=Matrix(*)  RndMeth=Zero
  Sum : Sum  Inputs=|+-
  Pk : Outport
  wires:
  Product3/1 -> Pk/1
  Mk/1 -> Product3/2
  Sum/1 -> Product3/1
  Product1/1 -> Sum/2
  Kk/1 -> Product1/1
  Hk/1 -> Product1/2
  Constant/1 -> Sum/1

== system ekffede/EKF/EKF_AHRS/Correction/Kalman Gain Matrix ==
  Mk : Inport
  Hk : Inport  Port=2
  Pqq : Inport  Port=3
  Math Function : Math  Operator=transpose  SaturateOnIntegerOverflow=on
  Product1 : Product  Multiplication=Matrix(*)  RndMeth=Zero
  Product2 : Product  Inputs=/  Multiplication=Matrix(*)  RndMeth=Zero
  Product3 : Product  Inputs=3  Multiplication=Matrix(*)  RndMeth=Zero
  Product4 : Product  Multiplication=Matrix(*)  RndMeth=Zero
  Sum : Sum  Inputs=|++
  Kk : Outport
  wires:
  Mk/1 -> Product1/1, Product3/2
  Hk/1 -> Math Function/1, Product3/1
  Math Function/1 -> Product1/2, Product3/3
  Product3/1 -> Sum/1
  Sum/1 -> Product2/1
  Product1/1 -> Product4/1
  Product2/1 -> Product4/2
  Pqq/1 -> Sum/2
  Product4/1 -> Kk/1

== system ekffede/EKF/EKF_AHRS/Correction/Kalman Gain Matrix (full) ==
  Mk : Inport
  Hk : Inport  Port=2
  Pqq : Inport  Port=3
  Math Function : Math  Operator=transpose  SaturateOnIntegerOverflow=on
  Product1 : Product  Multiplication=Matrix(*)  RndMeth=Zero
  Product2 : Product  Inputs=/  Multiplication=Matrix(*)  RndMeth=Zero
  Product3 : Product  Inputs=3  Multiplication=Matrix(*)  RndMeth=Zero
  Product4 : Product  Multiplication=Matrix(*)  RndMeth=Zero
  Sum : Sum  Inputs=|++
  Kk : Outport
  wires:
  Product4/1 -> Kk/1
  Product2/1 -> Product4/2
  Product1/1 -> Product4/1
  Sum/1 -> Product2/1
  Product3/1 -> Sum/1
  Math Function/1 -> Product3/3, Product1/2
  Hk/1 -> Product3/1, Math Function/1
  Mk/1 -> Product3/2, Product1/1
  Pqq/1 -> Sum/2

== system ekffede/EKF/EKF_AHRS/Correction/State Correction ==
  x_k : Inport
  zk : Inport  Port=2
  Kk : Inport  Port=3
  Product1 : Product  Multiplication=Matrix(*)  RndMeth=Zero
  Product2 : Product  Multiplication=Matrix(*)  RndMeth=Zero
  Subsystem : Subsystem
      mask Display: disp('h')
  Sum : Sum  Inputs=|-+
  Sum1 : Sum  Inputs=|++
  xk : Outport
  wires:
  Sum1/1 -> xk/1
  Product1/1 -> Sum1/1
  Sum/1 -> Product1/2
  zk/1 -> Sum/2
  Kk/1 -> Product1/1
  x_k/1 -> Sum1/2, Product2/2
  Product2/1 -> Sum/1
  Subsystem/1(Out1) -> Product2/1

== system ekffede/EKF/EKF_AHRS/Correction/Subsystem ==
  Matrix Concatenate : Concatenate  Mode=Multidimensional array  ConcatenateDimension=2
  R matrix : Constant  Value=eye(4)
  R matrix1 : Constant  Value=zeros(4,3)
  Out1 : Outport
  wires:
  R matrix/1 -> Matrix Concatenate/1
  R matrix1/1 -> Matrix Concatenate/2
  Matrix Concatenate/1 -> Out1/1

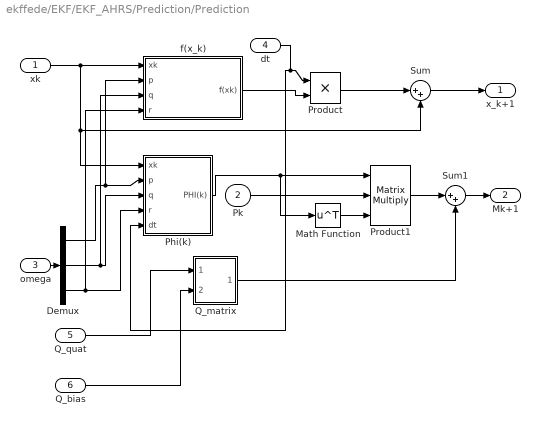
== system ekffede/EKF/EKF_AHRS/Prediction/Prediction ==
  xk : Inport
  Pk : Inport  Port=2
  omega : Inport  Port=3
  dt : Inport  Port=4
  Q_quat : Inport  Port=5
  Q_bias : Inport  Port=6
  Demux : Demux  Outputs=3
  Math Function : Math  Operator=transpose  SaturateOnIntegerOverflow=on
  Phi(k) : Subsystem
  Product : Product  RndMeth=Zero
  Product1 : Product  Inputs=3  Multiplication=Matrix(*)  RndMeth=Zero
  Q_matrix : Subsystem
      mask Display: disp('Q')
  Sum : Sum  Inputs=|++
  Sum1 : Sum  Inputs=|++
  f(x_k) : Subsystem
  x_k+1 : Outport
  Mk+1 : Outport  Port=2
  wires:
  Sum1/1 -> Mk+1/1
  Sum/1 -> x_k+1/1
  Product1/1 -> Sum1/1
  Math Function/1 -> Product1/3
  Pk/1 -> Product1/2
  Phi(k)/1(PHI(k)) -> Math Function/1, Product1/1
  Product/1 -> Sum/1
  f(x_k)/1(f(xk)) -> Product/2
  xk/1 -> Sum/2, Phi(k)/1(xk), f(x_k)/1(xk)
  Demux/1 -> Phi(k)/2(p), f(x_k)/2(p)
  Demux/2 -> f(x_k)/3(q), Phi(k)/3(q)
  Demux/3 -> Phi(k)/4(r), f(x_k)/4(r)
  omega/1 -> Demux/1
  Q_matrix/1(Out1) -> Sum1/2
  dt/1 -> Product/1, Phi(k)/5(dt)
  Q_quat/1 -> Q_matrix/1(Q_quat)
  Q_bias/1 -> Q_matrix/2(Q_bias)

== system ekffede/EKF/EKF_AHRS/Correction/State Correction/Subsystem ==
  Matrix Concatenate : Concatenate  Mode=Multidimensional array  ConcatenateDimension=2
  R matrix : Constant  Value=eye(4)
  R matrix1 : Constant  Value=zeros(4,3)
  Out1 : Outport
  wires:
  R matrix/1 -> Matrix Concatenate/1
  R matrix1/1 -> Matrix Concatenate/2
  Matrix Concatenate/1 -> Out1/1

== system ekffede/EKF/EKF_AHRS/Prediction/Prediction/Phi(k) ==
  xk : Inport
  p : Inport  Port=2
  q : Inport  Port=3
  r : Inport  Port=4
  dt : Inport  Port=5
  Constant2 : Constant  Value=eye(7)
  Product : Product  RndMeth=Zero
  Sum : Sum  Inputs=|++
  d f(x) / dx : Stateflow chart  TreatAsAtomicUnit=on
  PHI(k) : Outport
  wires:
  d f(x) / dx/1(F) -> Product/2
  xk/1 -> d f(x) / dx/1(x)
  Sum/1 -> PHI(k)/1
  Constant2/1 -> Sum/2
  Product/1 -> Sum/1
  p/1 -> d f(x) / dx/2(p)
  q/1 -> d f(x) / dx/3(q)
  r/1 -> d f(x) / dx/4(r)
  dt/1 -> Product/1

== system ekffede/EKF/EKF_AHRS/Prediction/Prediction/Q_matrix ==
  Q_quat : Inport
  Q_bias : Inport  Port=2
  " " : Constant  Value=zeros(4,3)
  " 1" : Constant  Value=zeros(3,4)
  MATLAB Function : Stateflow chart  TreatAsAtomicUnit=on
  MATLAB Function1 : Stateflow chart  TreatAsAtomicUnit=on
  Matrix Concatenate : Concatenate  Mode=Multidimensional array  ConcatenateDimension=2
  Matrix Concatenate1 : Concatenate  Mode=Multidimensional array  ConcatenateDimension=2
  Matrix Concatenate2 : Concatenate  Mode=Multidimensional array
  Out1 : Outport
  wires:
  " "/1 -> Matrix Concatenate/2
  Matrix Concatenate/1 -> Matrix Concatenate2/1
  " 1"/1 -> Matrix Concatenate1/1
  Matrix Concatenate1/1 -> Matrix Concatenate2/2
  Matrix Concatenate2/1 -> Out1/1
  MATLAB Function/1(y) -> Matrix Concatenate/1
  MATLAB Function1/1(y) -> Matrix Concatenate1/2
  Q_quat/1 -> MATLAB Function/1(Q_quat)
  Q_bias/1 -> MATLAB Function1/1(Q_bias)

== system ekffede/EKF/EKF_AHRS/Prediction/Prediction/f(x_k) ==
  xk : Inport
  p : Inport  Port=2
  q : Inport  Port=3
  r : Inport  Port=4
  Reshape : Reshape  OutputDimensionality=Column vector (2-D)
  "f(xk) " : Stateflow chart  TreatAsAtomicUnit=on
  f(xk) : Outport
  wires:
  "f(xk) "/1(dotxk) -> Reshape/1
  xk/1 -> "f(xk) "/1(x)
  Reshape/1 -> f(xk)/1
  r/1 -> "f(xk) "/4(r)
  q/1 -> "f(xk) "/3(q)
  p/1 -> "f(xk) "/2(p)

== matlab function EKF/QUEST_Pqq/q_matrix ==
  data: q1 input double; q_matrix output double; q2 input double; q3 input double; q4 input double
function q_matrix = fcn(q1,q2,q3,q4)

q_matrix=[ q4 -q3  q2 q1;
           q3  q4 -q1 q2;
          -q2  q1  q4 q3;
          -q1 -q2 -q3 q4];

== matlab function EKF/EKF_AHRS/Prediction/Prediction/Phi(k)/d f(x) / dx ==
  data: x input double; F output double; p input double; q input double; r input double
function F = fcn(x,p,q,r)
% This block supports the Embedded MATLAB subset.
% See the help menu for details. 

q1=x(1);
q2=x(2);
q3=x(3);
q0=x(4);
bp=x(5);
bq=x(6);
br=x(7);

F = [ 0,1/2*r-1/2*br,-1/2*q+1/2*bq,1/2*p-1/2*bp,-1/2*q0,1/2*q3,-1/2*q2;
       -1/2*r+1/2*br,0,1/2*p-1/2*bp,1/2*q-1/2*bq,-1/2*q3,-1/2*q0,1/2*q1;
       1/2*q-1/2*bq,-1/2*p+1/2*bp,0,1/2*r-1/2*br,1/2*q2,-1/2*q1,-1/2*q0;
       -1/2*p+1/2*bp,-1/2*q+1/2*bq,-1/2*r+1/2*br,0,1/2*q1,1/2*q2,1/2*q3;
       0,0,0,0,0,0,0;
       0,0,0,0,0,0,0;
       0,0,0,0,0,0,0];

== matlab function EKF/QUEST_Pqq/QUEST ==
  data: V1 input double; q_opt output double; V2 input double; W1 input double; W2 input double; PQQ output double; sig_acc input double; sig_m input double
function [q_opt,PQQ] = fcn(V1,V2,W1,W2,sig_acc,sig_m)

V1=V1/norm(V1);
V2=V2/norm(V2);
W1=W1/norm(W1);
W2=W2/norm(W2);

sig_quad_acc=sig_acc^2;
sig_quad_m=sig_m^2;
sig_quad_tot=1/(1/sig_quad_acc+1/sig_quad_m);
a1=sig_quad_tot/sig_quad_acc;
a2=sig_quad_tot/sig_quad_m;

cteta=dot(V1,V2)*dot(W1,W2)+(norm(cross(V1,V2)))*norm(cross(W1,W2));
lambda_max=sqrt(a1^2+a2^2+2*a1*a2*cteta);
S=a1*(W1*V1'+V1*W1')+ a2*(W2*V2'+V2*W2');
adjS=(det(S)*eye(3))/S;
sigma=0.5*sum(diag(S));
k=sum(diag(adjS));
delta=det(S);
Z=a1*cross(W1,V1)+ a2*cross(W2,V2);
alpha=lambda_max^2-sigma^2+k;
beta=lambda_max-sigma;
gamma=(lambda_max+sigma)*alpha-delta;

X=(alpha*eye(3)+beta*S+S*S)*Z;

q_opt = 1/sqrt(gamma^2+(norm(X))^2)*[X;gamma];

PQQ=1/4*(sig_quad_tot*eye(3)+(norm(cross(W1,W2)))^-2*((sig_quad_m-sig_quad_tot)*W1*W1'+(sig_quad_acc-sig_quad_tot)*W2*W2'+sig_quad_tot*dot(W1,W2)*(W1*W2'+W2*W1')));

== matlab function EKF/EKF_AHRS/Prediction/Prediction/f(x_k)/f(xk)  ==
  data: x input double; dotxk output double; p input double; q input double; r input double
function dotxk = fcn(x,p,q,r)
% This block supports the Embedded MATLAB subset.
% See the help menu for details. 

q1=x(1);
q2=x(2);
q3=x(3);
q0=x(4);
bp=x(5);
bq=x(6);
br=x(7);


dotxk=[0.5*q0*(p-bp)-0.5*q3*(q-bq)+0.5*q2*(r-br);
       0.5*q3*(p-bp)+0.5*q0*(q-bq)-0.5*q1*(r-br);
       -0.5*q2*(p-bp)+0.5*q1*(q-bq)+0.5*q0*(r-br);
       -0.5*q1*(p-bp)-0.5*q2*(q-bq)-0.5*q3*(r-br);
       0;
       0;
       0];

== matlab function dati/F,M./Embedded MATLAB Fx ==
  data: sfasamento input double; wave output double; ampiezza input double; frequenza input double; noise input double; t input double
function wave = fcn(sfasamento , ampiezza , frequenza,noise,t)
%#eml

wave = ampiezza*sin(sfasamento +2*pi*frequenza*t)+noise;

== matlab function dati/F,M./Embedded MATLAB Fy ==
  data: sfasamento input double; wave output double; ampiezza input double; frequenza input double; noise input double; t input double
function wave = fcn(sfasamento , ampiezza , frequenza,noise,t)
%#eml

wave = ampiezza*sin(sfasamento +2*pi*frequenza*t)+noise;

== matlab function dati/F,M./Embedded MATLAB Fz ==
  data: sfasamento input double; wave output double; ampiezza input double; frequenza input double; noise input double; t input double
function wave = fcn(sfasamento , ampiezza , frequenza,noise,t)
%#eml

wave = ampiezza*sin(sfasamento +2*pi*frequenza*t)+noise;

== matlab function dati/F,M./Embedded MATLAB pitch ==
  data: sfasamento input double; wave output double; ampiezza input double; frequenza input double; noise input double; t input double
function wave = fcn(sfasamento , ampiezza , frequenza,noise,t)
%#eml

wave = ampiezza*sin(sfasamento +2*pi*frequenza*t)+noise;

== matlab function dati/F,M./Embedded MATLAB roll ==
  data: sfasamento input double; wave output double; ampiezza input double; frequenza input double; noise input double; t input double
function wave = fcn(sfasamento , ampiezza , frequenza,noise,t)
%#eml

wave = ampiezza*sin(sfasamento +2*pi*frequenza*t)+noise;

== matlab function dati/F,M./Embedded MATLAB yaw ==
  data: sfasamento input double; wave output double; ampiezza input double; frequenza input double; noise input double; t input double
function wave = fcn(sfasamento , ampiezza , frequenza,noise,t)
%#eml

wave = ampiezza*sin(sfasamento +2*pi*frequenza*t)+noise;

== matlab function EKF/EKF_AHRS/Prediction/Prediction/Q_matrix/MATLAB Function ==
  data: Q_quat input double; y output double
function y = fcn(Q_quat)
%#codegen

y = diag(Q_quat);

== matlab function EKF/EKF_AHRS/Prediction/Prediction/Q_matrix/MATLAB Function1 ==
  data: Q_bias input double; y output double
function y = fcn(Q_bias)
%#codegen

y = diag(Q_bias);

== matlab function EKF/Gyro-bias ==
  data: gyro input double; gyrounbiased output double; bias input double
function gyrounbiased = fcn(gyro, bias)
%#codegen

gyrounbiased = [(gyro(1)-bias(1));
                (gyro(2)-bias(2));
                (gyro(3)-bias(3))];

== matlab function EKF/acc-cal ==
  data: acc_row input double; Acc_calibrate output double; acc_calibration input double
function Acc_calibrate = fcn(acc_row, acc_calibration)
%#codegen

acc_matrix = [acc_calibration(1),acc_calibration(2),acc_calibration(3);
                acc_calibration(4),acc_calibration(5),acc_calibration(6);
                acc_calibration(7),acc_calibration(8),acc_calibration(9)];
            
 acc_bias=[acc_calibration(10);
            acc_calibration(11);
            acc_calibration(12)];
        
 Acc_calibrate= acc_matrix*acc_row+acc_bias;

== matlab function EKF/mag-cal ==
  data: mag_row input double; mag_calibrate output double; mag_calibration input double
function mag_calibrate = fcn(mag_row, mag_calibration)
%#codegen

mag_matrix = [mag_calibration(1),mag_calibration(2),mag_calibration(3);
                mag_calibration(4),mag_calibration(5),mag_calibration(6);
                mag_calibration(7),mag_calibration(8),mag_calibration(9)];
            
 mag_bias=[mag_calibration(10);
            mag_calibration(11);
            mag_calibration(12)];
        
 mag_calibrate= mag_matrix*mag_row+mag_bias;
